simulink model "SchematyBlokoweSim"  (R2019a)
settings: Solver=VariableStepAuto  StartTime=0.0  StopTime=30  RelTol=1e-3
values from neighbouring files (symbols this model uses):
  k1 = 2    [SchematyBlokowe.m]    (also in TIPS_Lab_6_Zad_Dom.m = 0:N1-1)
  k2 = 2    [SchematyBlokowe.m]    (also in TIPS_Lab_6_Zad_Dom.m = 0:N2-1)
  T11 = 4    [SchematyBlokowe.m]
  T12 = 5    [SchematyBlokowe.m]
  T21 = 5    [SchematyBlokowe.m]
  T22 = 5    [SchematyBlokowe.m]
settings Model: Creator=ASUS_PEPE  LastModifiedBy=ASUS_PEPE

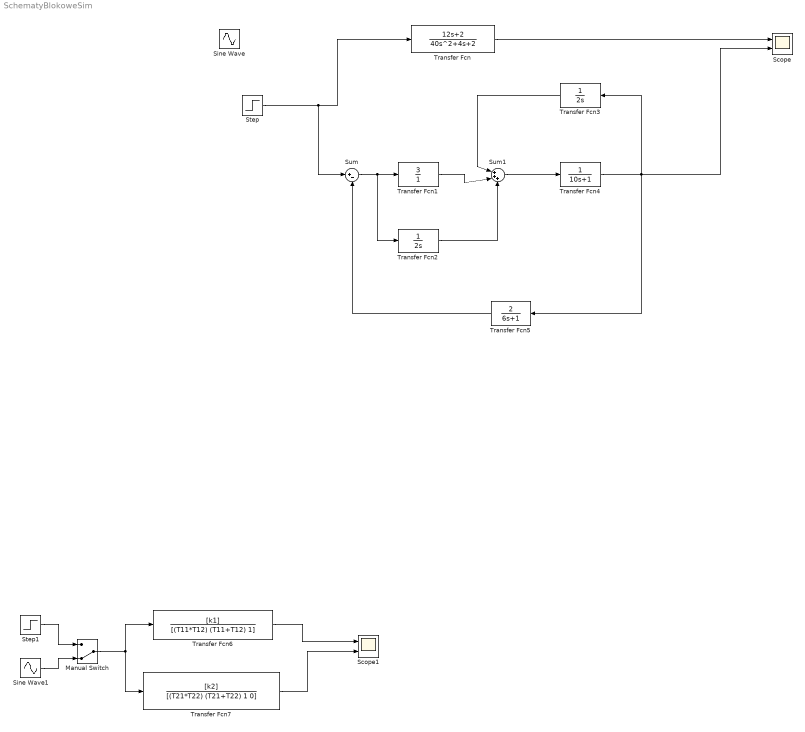
== system SchematyBlokoweSim ==
  Manual Switch : ManualSwitch  CurrentSetting=0
  Scope : Scope  NumInputPorts=2
  Scope1 : Scope  NumInputPorts=2
  Sine Wave : Sin  SampleTime=0
  Sine Wave1 : Sin  SampleTime=0
  Step : Step  SampleTime=0
  Step1 : Step  SampleTime=0
  Sum : Sum  Inputs=|+-
  Sum1 : Sum  Inputs=|+++
  Transfer Fcn : TransferFcn  Numerator=[12 2]  Denominator=[40 4 2]
  Transfer Fcn1 : TransferFcn  Numerator=[3]  Denominator=[1]
  Transfer Fcn2 : TransferFcn  Denominator=[2 0]
  Transfer Fcn3 : TransferFcn  Denominator=[2 0]
  Transfer Fcn4 : TransferFcn  Denominator=[10 1]
  Transfer Fcn5 : TransferFcn  Numerator=[2]  Denominator=[6 1]
  Transfer Fcn6 : TransferFcn  Numerator=[k1]  Denominator=[(T11*T12) (T11+T12) 1]
  Transfer Fcn7 : TransferFcn  Numerator=[k2]  Denominator=[(T21*T22) (T21+T22) 1 0]
  wires:
  Transfer Fcn/1 -> Scope/1
  Transfer Fcn5/1 -> Sum/2
  Sum/1 -> Transfer Fcn2/1, Transfer Fcn1/1
  Transfer Fcn1/1 -> Sum1/2
  Transfer Fcn2/1 -> Sum1/3
  Sum1/1 -> Transfer Fcn4/1
  Transfer Fcn3/1 -> Sum1/1
  Transfer Fcn4/1 -> Scope/2, Transfer Fcn5/1, Transfer Fcn3/1
  Step/1 -> Sum/1, Transfer Fcn/1
  Transfer Fcn6/1 -> Scope1/1
  Transfer Fcn7/1 -> Scope1/2
  Manual Switch/1 -> Transfer Fcn6/1, Transfer Fcn7/1
  Step1/1 -> Manual Switch/1
  Sine Wave1/1 -> Manual Switch/2
